simulink model "SimTrifasicoMeioLinha"  (R2021b)
settings: Solver=ode45  StartTime=0.0  StopTime=0.1  RelTol=1e-3  EnableMultiTasking=on
values from neighbouring files (symbols this model uses):
  C_matrix = [6.50686088743e-09  -1.1452177672e-10; -1.1452177672e-10  6.50686088743e-09]    [Modelo2fios2awg35.mat]
  dd = [60]    [RotinaCurtoCircuitoCompacto.m]    (also in RotinaCurtoCircuitoCompleta.m; RotinaCurtoCircuitoT2F_Trifasico.m)
  L_matrix = [0.00251001340283  0.000642378654137; 0.000642378654137  0.00251001340283]    [Modelo2fios2awg35.mat]
  m1 = n    [RotinaCurtoCircuitoCompacto.m]    (also in RotinaCurtoCircuitoCompleta.m; RotinaCurtoCircuitoT2F_Trifasico.m)
  m2 = 1 - m1    [RotinaCurtoCircuitoCompacto.m]    (also in RotinaCurtoCircuitoCompleta.m; RotinaCurtoCircuitoT2F_Trifasico.m)
  R_matrix = [1.15977689742  0.0575455112435; 0.0575455112435  1.15977689742]    [Modelo2fios2awg35.mat]
  RaTrif = 1e6    (= 1000000)    [RotinaCurtoCircuitoCompacto.m]    (also in RotinaCurtoCircuitoCompleta.m)
  RbTrif = 1e6    (= 1000000)    [RotinaCurtoCircuitoCompacto.m]    (also in RotinaCurtoCircuitoCompleta.m)
  RcTrif = 1e6    (= 1000000)    [RotinaCurtoCircuitoCompacto.m]    (also in RotinaCurtoCircuitoCompleta.m)
undefined symbols (not defined in the file or in its folder): D11, Delta
libraries: spsThreePhaseVIMeasurementLib x3, spsSeriesRLCBranchLib x3, spsDistributedParametersLineLib x2, spsThreePhaseTransformerTwoWindingsLib x2, spsThreePhaseSourceLib x1, spspowerguiLib x1
settings Model: Creator=laris  LastModifiedBy=USER
settings SolverCC: AlgebraicLoopSolver=TrustRegion
settings DataIOCC: LimitDataPoints=on  SaveFormat=Array  ReturnWorkspaceOutputs=off
settings OptimizationCC: LifeSpan=inf
settings DebuggingCC: SFUnexpectedBacktrackingDiag=warning  SFNoUnconditionalDefaultTransitionDiag=warning  SFExecutionAtInitializationDiag=none  SFMachineParentedDataDiag=warning  ArithmeticOperatorsInVariantConditions=warning
settings HardwareCC: ProdBitPerPointer=32  ProdBitPerSizeT=32  ProdBitPerPtrDiffT=32  ProdLargestAtomicFloat=None  ProdIntDivRoundTo=Undefined  ProdEndianess=Unspecified  ProdWordSize=32  ProdHWDeviceType=32-bit Generic
settings ModelReferenceCC: PropagateSignalLabelsOutOfModel=off
settings SFSimCC: SimUseLocalCustomCode=off  CustomCodeUndefinedFunction=UseInterfaceOnly
settings RTWCC: RTWUseLocalCustomCode=off
settings CodeAppCC: StateflowObjectComments=on
settings GRTTargetCC: TargetLangStandard=C89/C90 (ANSI)
settings ConfigComp: CovMetricSettings=dw  CovSaveCumulativeToWorkspaceVar=on  CovSaveSingleToWorkspaceVar=on  CovExternalEMLEnable=off
settings SimscapeCC: SimscapeNormalizeSystem=off

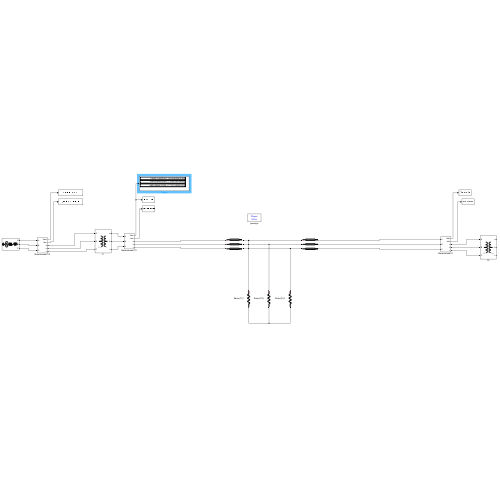
[thumbnail: Simulink's stored preview of the top-level diagram]
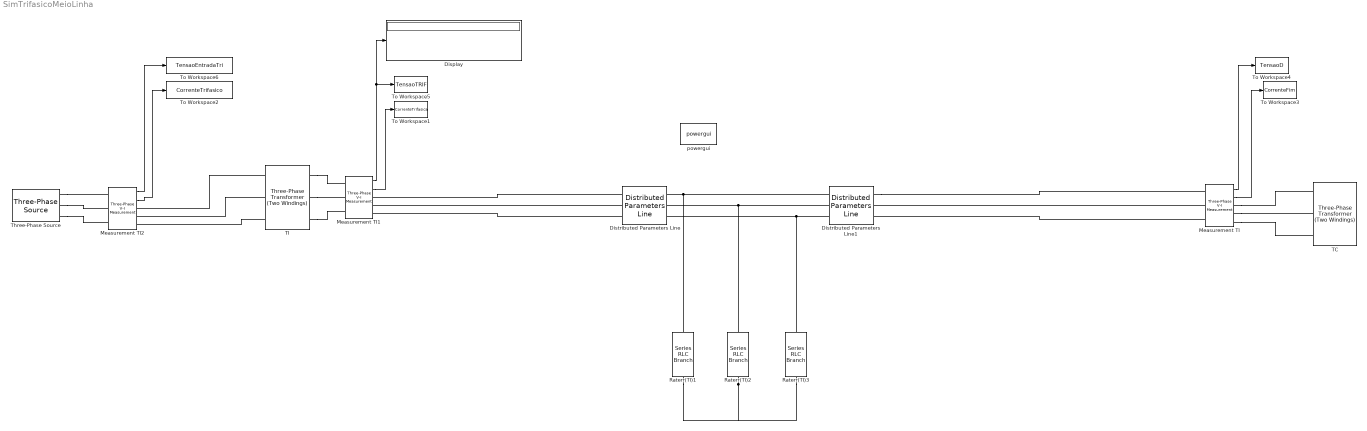
== system SimTrifasicoMeioLinha ==
  Display : Display
  Distributed Parameters Line : spsDistributedParametersLineLib/Distributed Parameters Line  Phases=3  Length=dd * m1  Frequency=60  Resistance=R_matrix  Inductance=L_matrix  Capacitance=C_matrix  x1=[1304.44069459451 13976.1540670455 13971.5913636337;376.991118430775 376.991118430775 376.991118430775;-2.72384421214701 -1.12771418755211 -2.69949152347311]  x2=[1310.63312555978 14015.3156095758 14011.0617932711;376.991118430775 376.991118430775 376.991118430775;-2.72720266013493 -1.13468561873066 -2.70773972547183]  x3=[1.09667432232134 33.381660203175 38.4309145640101;376.991118430775 376.991118430775 376.991118430775;-2.82342685780924 -1.20807333972374 -2.78088181487407]  x4=[1.09853756573713 33.4347126878563 38.4840313697474;376.991118430775 376.991118430775 376.991118430775;-2.72740448710286 -1.13489212505125 -2.70790405802449]  x5=0.000260094822325124  V1=ones(3,3)  V2=ones(3,3)  I1=ones(3,3)  I2=ones(3,3)  nHarmo=1  Measurements=None  Decoupling=on  VsMag0=[11175.6153395108 11940.2648952892 11174.6307421375]  VrMag0=[11215.4202070305 11975.5170963021 11196.2287691596]  VsAngle0=[-32.3718705303 -150.249697348215 91.9694998461809]  VrAngle0=[-32.8017780856475 -150.703771725416 91.5514176383415]  IsMag0=[31.2669397325685 34.7573534664733 31.2418111355644]  IrMag0=[31.3295094400185 34.8057687533619 31.2740551638241]  IsAngle0=[-30.5540771763404 -154.923675569618 80.9145071553585]  IrAngle0=[-26.3860525940854 -150.716449742827 85.094678273751]
      settings: SourceProductBaseCode=PS
  Distributed Parameters Line1 : spsDistributedParametersLineLib/Distributed Parameters Line  Phases=3  Length=dd * m2  Frequency=60  Resistance=R_matrix  Inductance=L_matrix  Capacitance=C_matrix  x1=[1310.63312555978 14015.3156095758 14011.0617932711;376.991118430775 376.991118430775 376.991118430775;-2.62924737375808 -1.05773417928016 -2.63043438306304]  x2=[1310.6330561365 14015.3143476049 14011.0605732421;376.991118430775 376.991118430775 376.991118430775;-2.62924739925307 -1.05773416740828 -2.63043436787328]  x3=[1.15339748819258 38.1828514509477 45.017388130895;376.991118430775 376.991118430775 376.991118430775;-2.62904908831067 -1.05753632280468 -2.63027816484447]  x4=[1.15438632790488 38.2132910748968 45.0478878496462;376.991118430775 376.991118430775 376.991118430775;-2.62954362598914 -1.05800894469494 -2.63066791848513]  x5=2.60355177502627e-07  V1=ones(3,3)  V2=ones(3,3)  I1=ones(3,3)  I2=ones(3,3)  nHarmo=1  Measurements=None  Decoupling=on  VsMag0=[11215.4202070305 11975.5170963021 11196.2287691596]  VrMag0=[11215.419150672 11975.5160805828 11196.2277984663]  VsAngle0=[-32.8017780856475 -150.703771725416 91.5514176383415]  VrAngle0=[-32.8017773361158 -150.703771009203 91.5514184758037]  IsMag0=[32.795758520322 36.5889728471396 32.7349170770078]  IrMag0=[32.8192531259242 36.6138870674152 32.7610172159657]  IsAngle0=[-26.1214525499856 -150.698041933584 84.8724229409834]  IrAngle0=[-26.1503008046441 -150.720486787229 84.8503062133126]
      settings: SourceProductBaseCode=PS
  Measurement TI : spsThreePhaseVIMeasurementLib/Three-Phase V-I Measurement  VoltageMeasurement=phase-to-phase  SetLabelV=off  LabelV=Vabc  Vpu=off  VpuLL=off  CurrentMeasurement=yes  SetLabelI=off  LabelI=Iabc  Ipu=off  Pbase=100e6  Vbase=500e3  OutputType=Magnitude  PhasorSimulation=on  PSBequivalent=0
  Measurement TI1 : spsThreePhaseVIMeasurementLib/Three-Phase V-I Measurement  VoltageMeasurement=phase-to-phase  SetLabelV=off  LabelV=Vabc  Vpu=off  VpuLL=off  CurrentMeasurement=yes  SetLabelI=off  LabelI=Iabc  Ipu=off  Pbase=100e6  Vbase=500e3  OutputType=Complex  PhasorSimulation=on  PSBequivalent=0
  Measurement TI2 : spsThreePhaseVIMeasurementLib/Three-Phase V-I Measurement  VoltageMeasurement=phase-to-phase  SetLabelV=off  LabelV=Vabc  Vpu=off  VpuLL=off  CurrentMeasurement=yes  SetLabelI=off  LabelI=Iabc  Ipu=off  Pbase=100e6  Vbase=500e3  OutputType=Magnitude  PhasorSimulation=on  PSBequivalent=0
  Raterr(TI)1 : spsSeriesRLCBranchLib/Series RLC Branch  LConnTagsString=__new0  RConnTagsString=__new0  BranchType=R  Resistance=RaTrif  Inductance=0  SetiL0=off  InitialCurrent=0  Capacitance=1e-6  Setx0=off  InitialVoltage=0  Measurements=None
  Raterr(TI)2 : spsSeriesRLCBranchLib/Series RLC Branch  LConnTagsString=__new0  RConnTagsString=__new0  BranchType=R  Resistance=RbTrif  Inductance=0  SetiL0=off  InitialCurrent=0  Capacitance=1e-6  Setx0=off  InitialVoltage=0  Measurements=None
  Raterr(TI)3 : spsSeriesRLCBranchLib/Series RLC Branch  LConnTagsString=__new0  RConnTagsString=__new0  BranchType=R  Resistance=RcTrif  Inductance=0  SetiL0=off  InitialCurrent=0  Capacitance=1e-6  Setx0=off  InitialVoltage=0  Measurements=None
  TC : spsThreePhaseTransformerTwoWindingsLib/Three-Phase Transformer (Two Windings)  Winding1Connection=Delta (D11)  Winding2Connection=Yg  CoreType=Three single-phase transformers  SetSaturation=off  Hysteresis=off  DataFile='hysteresis'  SetInitialFlux=off  Measurements=None  UNITS=pu  NominalPower=[120e3 , 60]  Winding1=[13800 0.0048118 0.018511]  Winding2=[380 0.0048119 0.018511]  Rm=5.801193266567229e+02  Lm=8.409977380031759e+02  L0=0.50001  Saturation=[0 0;0.0012545 0.01913;0.52272 0.024231]  InitialFluxes=[0.66025 -0.66025 0.57768]  BreakLoop=off  DiscreteSolver=Trapezoidal iterative  DataType=off  TransfoNumber=1
  TI : spsThreePhaseTransformerTwoWindingsLib/Three-Phase Transformer (Two Windings)  Winding1Connection=Delta (D11)  Winding2Connection=Y  CoreType=Three single-phase transformers  SetSaturation=off  Hysteresis=off  DataFile='hysteresis'  SetInitialFlux=off  Measurements=All measurements (V I Fluxes)  UNITS=pu  NominalPower=[120e3 , 60 ]  Winding1=[13800 0.0048119 0.018511]  Winding2=[13800 0.0048119 0.018511]  Rm=1.730769230769231e+03*1000  Lm=40.010686750359440*1000  L0=6.3145  Saturation=[0 0;0.0012545 0.01913;0.52272 0.024231]  InitialFluxes=[34.179 -34.179 29.906]  BreakLoop=off  DiscreteSolver=Trapezoidal iterative  DataType=off  TransfoNumber=1
  Three-Phase Source : spsThreePhaseSourceLib/Three-Phase Source  InternalConnection=Yg  VoltagePhases=off  Voltage=13.8e3  PhaseAngle=0  Voltage_phases=[25e3 25e3 25e3]/sqrt(3)  PhaseAngles_phases=[0 -120 +120]  Frequency=60  NonIdealSource=on  SpecifyImpedance=on  Resistance=0.8929  Inductance=16.58e-3  ShortCircuitLevel=120e6  BaseVoltage=13.8e3  XRratio=7  BusType=swing  Pref=10e3  Qref=0  Prefabc=[10e3, 10e3, 10e3]  Qrefabc=[0, 0, 0]  Qmin=-inf  Qmax=inf
  To Workspace1 : ToWorkspace  VariableName=CorrenteTrifasica  SampleTime=-1
      settings: MaxDataPoints=1
  To Workspace2 : ToWorkspace  VariableName=CorrenteTrifasico  SampleTime=-1
      settings: MaxDataPoints=1
  To Workspace3 : ToWorkspace  VariableName=CorrenteFim  SampleTime=-1
      settings: MaxDataPoints=1
  To Workspace4 : ToWorkspace  VariableName=TensaoD  SampleTime=-1
      settings: MaxDataPoints=1
  To Workspace5 : ToWorkspace  VariableName=TensaoTRIF  SampleTime=-1
      settings: MaxDataPoints=1
  To Workspace6 : ToWorkspace  VariableName=TensaoEntradaTri  SampleTime=-1
      settings: MaxDataPoints=1
  powergui : spspowerguiLib/powergui  Priority=1  SimulationMode=Phasor  SampleTime=50e-6  frequency=60  Iterations=50  frequencyindice=60  Pbase=100e6  ErrMax=1e-4  UnitsV=kV  UnitsW=MW  buscounter=0  FunctionMessages=off  echomessages=off  EnableUseOfTLC=off  CurrentSourceSwitches=off  DisableSnubberDevices=off  DisableRonSwitches=off  DisableVfSwitches=off  DisplayEquations=off  AutomaticDiscreteSolvers=off  SolverType=Tustin/Backward Euler (TBE)  Interpol=off  ExternalGateDelay=off  methode=off  Ts=100  x0status=blocks  SPID=on  SwTol=0  HookPort=off  NonlinearTolerance=1e-4  nMaxIteration=100  ContinueOnMaxIteration=off  RestoreLinks=warning  ResistiveCurrentMeasurement=off  Frange=[0:2:500]  Ylog=off  Xlog=on  ShowGrid=off  save=off  variable=ZData  structure=0  ZoomFFT=off  StartTime=0.0  cycles=1  DisplayStyle=1  fundamental=60  FreqAxis=off  MaxFrequency=1000  frequencyindicesteady=1  RmsSteady=1  display=off
  wires:
  Measurement TI/1 -> To Workspace4/1
  Measurement TI1/2 -> To Workspace1/1
  Measurement TI1/1 -> Display/1, To Workspace5/1
  Measurement TI2/1 -> To Workspace6/1
  Measurement TI2/2 -> To Workspace2/1
  Measurement TI/2 -> To Workspace3/1
  connections:
  Distributed Parameters Line1/LConn2 -- Raterr(TI)2/LConn1 -- Distributed Parameters Line/RConn2
  Measurement TI/RConn1 -- TC/LConn1
  Measurement TI/RConn2 -- TC/LConn2
  Measurement TI/RConn3 -- TC/LConn3
  TI/RConn2 -- Measurement TI1/LConn2
  TI/RConn1 -- Measurement TI1/LConn1
  Distributed Parameters Line/LConn3 -- Measurement TI1/RConn3
  Distributed Parameters Line1/LConn3 -- Raterr(TI)3/LConn1 -- Distributed Parameters Line/RConn3
  TI/RConn3 -- Measurement TI1/LConn3
  Three-Phase Source/RConn3 -- Measurement TI2/LConn3
  Three-Phase Source/RConn2 -- Measurement TI2/LConn2
  Three-Phase Source/RConn1 -- Measurement TI2/LConn1
  TI/LConn1 -- Measurement TI2/RConn1
  TI/LConn2 -- Measurement TI2/RConn2
  TI/LConn3 -- Measurement TI2/RConn3
  Distributed Parameters Line/LConn1 -- Measurement TI1/RConn1
  Distributed Parameters Line/LConn2 -- Measurement TI1/RConn2
  Distributed Parameters Line1/LConn1 -- Raterr(TI)1/LConn1 -- Distributed Parameters Line/RConn1
  Raterr(TI)2/RConn1 -- Raterr(TI)1/RConn1 -- Raterr(TI)3/RConn1
  Measurement TI/LConn3 -- Distributed Parameters Line1/RConn3
  Measurement TI/LConn2 -- Distributed Parameters Line1/RConn2
  Distributed Parameters Line1/RConn1 -- Measurement TI/LConn1
